simulink model "Phone_B"  (R2020a)
settings: Solver=FixedStepAuto  StartTime=0.0  StopTime=inf  RelTol=1e-3
undefined symbols (not defined in the file): a, Audio_Receive, Lat, Latitude_Receive, Lon, Longitude_Receive, TCP
libraries: androidcommunicationlib x3, androidaudiovideolib x2, androiduilib x2
settings Model: Creator=Hrriday  LastModifiedBy=Hrriday
settings OptimizationCC: EnhancedBackFolding=on  PassReuseOutputArgsAs=Individual arguments  ZeroExternalMemoryAtStartup=off  ZeroInternalMemoryAtStartup=off  MaxStackSize=64  OptimizeBlockOrder=speed  DifferentSizesBufferReuse=on  OptimizationCustomize=off  EfficientTunableParamExpr=on
settings DebuggingCC: ParameterTunabilityLossMsg=error
settings HardwareCC: ProdBitPerPointer=32  ProdBitPerSizeT=32  ProdBitPerPtrDiffT=32  ProdLargestAtomicInteger=Long  ProdLargestAtomicFloat=Double  ProdWordSize=32  ProdHWDeviceType=ARM Compatible->ARM Cortex
settings SFSimCC: MATLABDynamicMemAlloc=off
settings RTWCC: SystemTargetFile=ert.tlc  HardwareBoard=Android Device  TemplateMakefile=ert_default_tmf  RTWVerbose=off  Toolchain=Android SDK/NDK Tools
settings CodeAppCC: ForceParamTrailComments=on  IgnoreCustomStorageClasses=off  OperatorAnnotations=on  SimulinkDataObjDesc=on  SFDataObjDesc=on  InsertBlockDesc=on

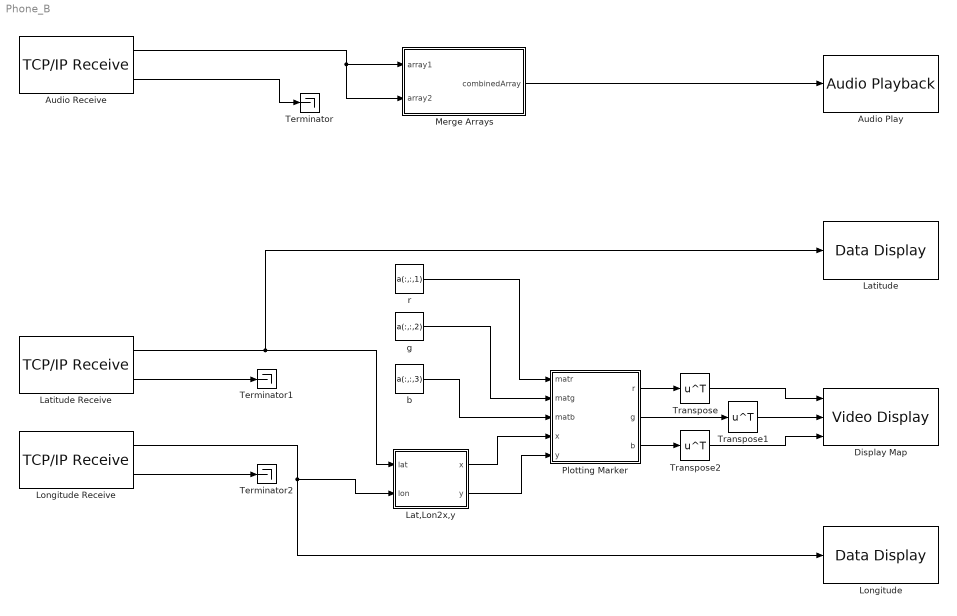
== system Phone_B ==
  Audio Play : androidaudiovideolib/Audio Playback  SampleFreq=24000  AudioSamplingFreq=24000  SampleTime=0.1  DeviceStr=0  QueueDuration=0  BlockPlatform=Android
      settings: SourceProductBaseCode=ANDROID
  Audio Receive : androidcommunicationlib/TCP//IP Receive  TCPReceiveId=TCP/Audio_Receive  Mode_=Client  LocalServerPort_=25000  RemoteAddr_=10.7.18.113  RemoteServerPort_=25000  DataType_=int16  DataSize_=2400  SampleTime_=0.1  SimulateUsing=Code generation  ClientPortBindingSelection_=off  ClientPortToBind_=35000  BlockingMode_=off  BlockTimeout_=0.1
      settings: SourceProductBaseCode=ANDROID
  Display Map : androidaudiovideolib/Video Display  BlockPlatform=Android
      settings: SourceProductBaseCode=ANDROID
  Lat,Lon2x,y : MATLAB Function  TreatAsAtomicUnit=on
  Latitude : androiduilib/Data Display  DataDisplayId=TCP/Lat  Format=Float  Precision=6  SimulateUsing=Code generation  blockPlatform=Android
      settings: SourceProductBaseCode=ANDROID
  Latitude Receive : androidcommunicationlib/TCP//IP Receive  TCPReceiveId=TCP/Latitude_Receive  Mode_=Client  LocalServerPort_=25000  RemoteAddr_=10.7.18.113  RemoteServerPort_=22500  DataType_=double  DataSize_=1  SampleTime_=2  SimulateUsing=Code generation  ClientPortBindingSelection_=off  ClientPortToBind_=35000  BlockingMode_=off  BlockTimeout_=0.1
      settings: SourceProductBaseCode=ANDROID
  Longitude : androiduilib/Data Display  DataDisplayId=TCP/Lon  Format=Float  Precision=6  SimulateUsing=Code generation  blockPlatform=Android
      settings: SourceProductBaseCode=ANDROID
  Longitude Receive : androidcommunicationlib/TCP//IP Receive  TCPReceiveId=TCP/Longitude_Receive  Mode_=Client  LocalServerPort_=25000  RemoteAddr_=10.7.18.113  RemoteServerPort_=20000  DataType_=double  DataSize_=1  SampleTime_=2  SimulateUsing=Code generation  ClientPortBindingSelection_=off  ClientPortToBind_=35000  BlockingMode_=off  BlockTimeout_=0.1
      settings: SourceProductBaseCode=ANDROID
  Merge Arrays : MATLAB Function  TreatAsAtomicUnit=on
  Plotting Marker : MATLAB Function  TreatAsAtomicUnit=on
  Terminator : Terminator
  Terminator1 : Terminator
  Terminator2 : Terminator
  Transpose : Math  Operator=transpose  SaturateOnIntegerOverflow=on
  Transpose1 : Math  Operator=transpose  SaturateOnIntegerOverflow=on
  Transpose2 : Math  Operator=transpose  SaturateOnIntegerOverflow=on
  b : Constant  Value=a(:,:,3)  VectorParams1D=off  OutDataTypeStr=uint8
  g : Constant  Value=a(:,:,2)  VectorParams1D=off  OutDataTypeStr=uint8
  r : Constant  Value=a(:,:,1)  VectorParams1D=off  OutDataTypeStr=uint8
  wires:
  Audio Receive/1 -> Merge Arrays/2(array2), Merge Arrays/1(array1)
  Merge Arrays/1(combinedArray) -> Audio Play/1
  Audio Receive/2 -> Terminator/1
  r/1 -> Plotting Marker/1(matr)
  g/1 -> Plotting Marker/2(matg)
  b/1 -> Plotting Marker/3(matb)
  Plotting Marker/1(r) -> Transpose/1
  Plotting Marker/2(g) -> Transpose1/1
  Plotting Marker/3(b) -> Transpose2/1
  Lat,Lon2x,y/1(x) -> Plotting Marker/4(x)
  Lat,Lon2x,y/2(y) -> Plotting Marker/5(y)
  Transpose/1 -> Display Map/1
  Transpose1/1 -> Display Map/2
  Transpose2/1 -> Display Map/3
  Longitude Receive/1 -> Longitude/1, Lat,Lon2x,y/2(lon)
  Longitude Receive/2 -> Terminator2/1
  Latitude Receive/2 -> Terminator1/1
  Latitude Receive/1 -> Lat,Lon2x,y/1(lat), Latitude/1

== matlab function Phone_B/Lat,Lon2x,y ==
  data: lat input; x output; y output; lon input
function [x,y] = fcn(lat,lon)
Lat0 = 23.2089;
Lon0 = 72.6833;
if lat == 0 && lon == 0
    lat = Lat0;
    lon = Lon0;
end
Lat1 = 23.2111;
Lon1 = 72.6858;
r = 460;
c = 460;

y = (lon-Lon0)/(Lon1-Lon0)*c;
x = 460 - (lat-Lat0)/(Lat1-Lat0)*r;
end

== matlab function Phone_B/Merge Arrays ==
  data: array1 input; combinedArray output; array2 input
function combinedArray = pairArrays(array1,array2)
    combinedArray = [array1(:),array2(:)];
end

== matlab function Phone_B/Plotting Marker ==
  data: matr input; matg input; matb input; r output; g output; b output; x input; y input
function [r,g,b] = fcn(matr,matg,matb,x,y)
for i = x-7:x+7
    for j = y-7:y+7
        matr(i,j,1) = 200;
        matb(i,j,1) = 0;
        matg(i,j,1) = 0;
    end
end

r = matr;
g = matg;
b = matb;
end
